simulink model "asbCubeSat"  (R2021a)
settings: Solver=FixedStepAuto  StartTime=0.0  StopTime=43200  FixedStep=CubeSatTimeStep  RelTol=1e-3  EnableMultiTasking=on
PreLoadFcn:
  | if ~builtin('license','test','Virtual_Reality_Toolbox')
  |     assignin('base','variantVisualization',0)
  | end
InitFcn:
  | if evalin('base', 'exist(''variantVisualization'',''var'')') && ...
  |         evalin('base', 'variantVisualization == 1')
  |     if ~builtin('license','checkout','Virtual_Reality_Toolbox')
  |         error(message('aeroblks_cubesat:cubesat:licenseFailAnim'));
  |     end
  | end
  | 
  | if ~evalin('base','exist(''CubeSatTimeStep'')')
  |     assignin('base','CubeSatTimeStep',5);
  | end
undefined symbols (not defined in the file): asbCubeSatEnvironmentLib, CubeSatTimeStep, Enviroment, IAU, initCond, km, s, vehicle
libraries: aerolibutil x17, sharedutil x6, aerolibconvert2 x4, aerolibtransform2 x1, aerolibcelestial x1, SignalEditorBlockLib x1, asbCubeSatSensorsLib x1, asbCubeSatDynamicsLib x1, aerolibobsolete x1, aerolibattitudesys x1, simulink x1, vrlib x1
settings Model: RequirementInfo={} %GIDa_aedc6be2_fb6a_446c_8c25_10b8bc9db182  SnapshotInterval=1  ExtModeAutoUpdateStatusClock=off  OrderedModelArguments=off  Creator=The MathWorks, Inc.  LastModifiedBy=noraw
settings SolverCC: AlgebraicLoopSolver=TrustRegion
settings DataIOCC: LimitDataPoints=on  SaveFormat=Array  SaveOutput=off  DSMLogging=off  SaveTime=off  ReturnWorkspaceOutputs=off
settings OptimizationCC: DefaultParameterBehavior=Inlined  OptimizeBlockIOStorage=off  BufferReuse=off  GlobalBufferReuse=off  ExpressionFolding=off  ExpressionDepthLimit=2147483647  LocalBlockOutputs=off  InitFltsAndDblsToZero=on  LifeSpan=inf  OptimizeDataStoreBuffers=off  BusAssignmentInplaceUpdate=off
settings DebuggingCC: SignalResolutionControl=TryResolveAllWithWarning  MultiTaskDSMMsg=warning  MultiTaskCondExecSysMsg=none  AssertControl=DisableAll  StateNameClashWarn=warning  PregeneratedLibrarySubsystemCodeDiagnostic=none  SFUnexpectedBacktrackingDiag=warning  SFNoUnconditionalDefaultTransitionDiag=warning  SFExecutionAtInitializationDiag=none  SFMachineParentedDataDiag=warning  ArithmeticOperatorsInVariantConditions=warning
settings HardwareCC: ProdBitPerPointer=32  ProdBitPerSizeT=32  ProdBitPerPtrDiffT=32  ProdLargestAtomicFloat=None  ProdIntDivRoundTo=Undefined  ProdEndianess=Unspecified  ProdWordSize=32  ProdHWDeviceType=32-bit Generic
settings ModelReferenceCC: UpdateModelReferenceTargets=IfOutOfDate  ModelReferenceMinAlgLoopOccurrences=on  PropagateSignalLabelsOutOfModel=off
settings SFSimCC: SimUseLocalCustomCode=off
settings RTWCC: RTWUseLocalCustomCode=off
settings CodeAppCC: StateflowObjectComments=on
settings GRTTargetCC: TargetFcnLib=ansi_tfl_tmw.mat  TargetLangStandard=C89/C90 (ANSI)  CombineOutputUpdateFcns=off  GRTInterface=on
settings ConfigComp: CovMetricSettings=dw  CovSaveCumulativeToWorkspaceVar=on  CovSaveSingleToWorkspaceVar=on  CovExternalEMLEnable=off

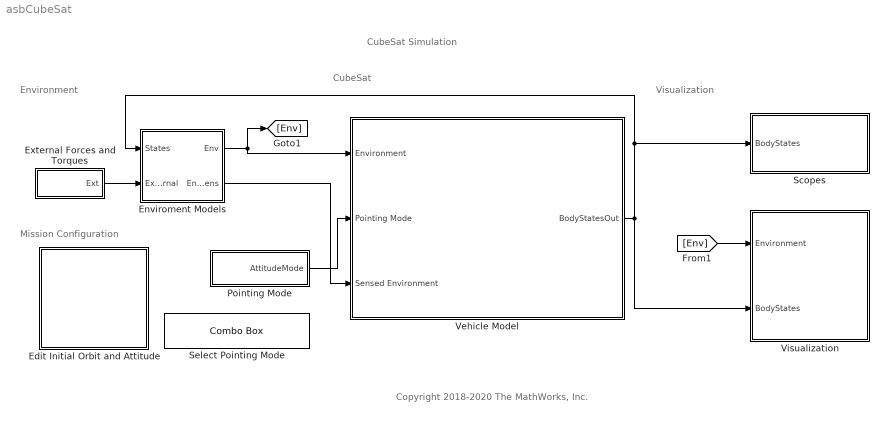
== system asbCubeSat ==
  note: Visualization
  note: CubeSat
  note: Environment
  note: Copyright 2018-2020 The MathWorks, Inc.
  note: CubeSat Simulation
  note: Mission Configuration
  Edit Initial Orbit and Attitude : Subsystem  mask(CubeSat Initial Conditions){sim_t0=2458488, epoch=2451545, method=Keplerian Orbital Elements, a=6786233.13, ecc=0.0010537, incl=51.7519, omega=95.2562, argp=93.4872, nu=302.9234, truelon=0, arglat=0, lonper=0, r_eci=[-2981784.257 5207055.9381 3161595.3068], v_eci=[-3384.4834 -4887.7595 4843.4609], r_ecef=[-5762650.9114 -1682704.282 3156028.2879], v_ecef=[3832.57 -4024.9014 4837.4311], lla=[27.88080034 -163.722102 408851.6223], v_ned=[5468.7396 4937.8129 -7.4627367], euler=[0 0 0], pqr=[0 0 -0.05168]}
      mask prompts: sim_t0 "spacecraft:cubesat:StartDate"; epoch "spacecraft:cubesat:ECIEpoch"; method "spacecraft:cubesat:InputMethod"; a "spacecraft:cubesat:SemiMajorAxis"; ecc "spacecraft:cubesat:Eccentricity"; incl "spacecraft:cubesat:Inclination"; omega "spacecraft:cubesat:RAAN"; argp "spacecraft:cubesat:ArgP"; nu "spacecraft:cubesat:TrueAnomaly"; truelon "spacecraft:cubesat:TrueLon"; arglat "spacecraft:cubesat:ArgLat"; lonper "spacecraft:cubesat:LonPer"; r_eci "spacecraft:cubesat:ECIPos"; v_eci "spacecraft:cubesat:ECIVel"; r_ecef "spacecraft:cubesat:ECEFPos"; v_ecef "spacecraft:cubesat:ECEFVel"; lla "spacecraft:cubesat:LLA"; v_ned "spacecraft:cubesat:NEDVel"; euler "spacecraft:cubesat:Euler"; pqr "spacecraft:cubesat:BodyAngRates"
      mask help: spacecraft:cubesat:InitCondBlockDesc
      mask init:
      | initCond = cubeSatCallback(gcb, 'computeIC', method, sim_t0, epoch, a, ecc, incl,...
      |     omega, argp, nu, truelon, arglat, lonper, r_eci, v_eci, r_ecef, v_ecef, lla,...
      |     v_ned, euler, pqr);
      mask TypeOptions method: spacecraft:cubesat:InputKeplerian | spacecraft:cubesat:InputECI | spacecraft:cubesat:InputECEF | spacecraft:cubesat:InputLLANED
      mask Callback method: cubeSatCallback(gcb, 'handleMethod');
      mask Callback ecc: cubeSatCallback(gcb, 'handleCircularOrbit');
      mask Callback incl: cubeSatCallback(gcb, 'handleCircularOrbit');
      mask DialogControl sim_t0 Prompt: Start date [Julian date]:
      mask DialogControl sim_t0 Tooltip: spacecraft:spacecraft:StartDateTT
      mask DialogControl icTab Prompt: spacecraft:cubesat:InitCond
      mask DialogControl epoch Prompt: Epoch of ECI frame [Julian date]:
      mask DialogControl epoch Tooltip: spacecraft:cubesat:ECIEpochTT
      mask DialogControl Container9 Prompt: spacecraft:cubesat:InitCondOrbit
      mask DialogControl method Prompt: Input method:
      mask DialogControl method Tooltip: spacecraft:cubesat:InputMethodTT
      mask DialogControl a Prompt: Semi-major axis [m]:
      mask DialogControl a Tooltip: spacecraft:cubesat:SemiMajorAxisTT
      mask DialogControl ecc Prompt: Eccentricity:
      mask DialogControl ecc Tooltip: spacecraft:cubesat:EccentricityTT
      mask DialogControl incl Prompt: Inclination [deg]:
      mask DialogControl incl Tooltip: spacecraft:cubesat:InclinationTT
      mask DialogControl omega Prompt: Right ascension of the ascending node [deg]:
      mask DialogControl omega Tooltip: spacecraft:cubesat:RAANTT
      mask DialogControl argp Prompt: Argument of periapsis [deg]:
      mask DialogControl argp Tooltip: spacecraft:cubesat:ArgPTT
      mask DialogControl nu Prompt: True anomaly [deg]:
      mask DialogControl nu Tooltip: spacecraft:cubesat:TrueAnomalyTT
      mask DialogControl truelon Prompt: True longitude [deg] (circular equatorial):
      mask DialogControl truelon Tooltip: spacecraft:cubesat:TrueLonTT
      mask DialogControl arglat Prompt: Argument of latitude [deg] (circular inclined):
      mask DialogControl arglat Tooltip: spacecraft:cubesat:ArgLatTT
      mask DialogControl lonper Prompt: Longitude of periapsis [deg] (elliptical equatorial):
      mask DialogControl lonper Tooltip: spacecraft:cubesat:LonPerTT
      mask DialogControl r_eci Prompt: ECI position vector [m]:
      mask DialogControl r_eci Tooltip: spacecraft:cubesat:ECIPosTT
      mask DialogControl v_eci Prompt: ECI velocity vector [m/s]:
      mask DialogControl v_eci Tooltip: spacecraft:cubesat:ECIVelTT
      mask DialogControl r_ecef Prompt: ECEF position vector [m]:
      mask DialogControl r_ecef Tooltip: spacecraft:cubesat:ECEFPosTT
      mask DialogControl v_ecef Prompt: ECEF velocity vector [m/s]:
      mask DialogControl v_ecef Tooltip: spacecraft:cubesat:ECEFVelTT
      mask DialogControl lla Prompt: Geodetic latitude, longitude, altitude [deg, deg, m]:
      mask DialogControl lla Tooltip: spacecraft:cubesat:LLATT
      mask DialogControl v_ned Prompt: NED velocity vector [m/s]:
      mask DialogControl v_ned Tooltip: spacecraft:cubesat:NEDVelTT
      mask DialogControl Container11 Prompt: spacecraft:cubesat:InitCondAttitude
      mask DialogControl euler Prompt: Initial Euler angles (roll, pitch, yaw) [deg]:
      mask DialogControl euler Tooltip: spacecraft:cubesat:EulerTT
      mask DialogControl pqr Prompt: Initial body angular rates [deg/s]:
      mask DialogControl pqr Tooltip: spacecraft:cubesat:BodyAngRatesTT
      mask Display:
      | text(.1, .9, [' a = ' sprintf('%.1f', str2double(get_param(gcb, 'a'))) ' m'],'horizontalAlignment','left','texmode','on');
      | text(.1, .75, [' e = ' get_param(gcb, 'ecc')],'horizontalAlignment','left','texmode', 'on')
      | text(.1, .6, ['  i = ' get_param(gcb, 'incl') '\circ'],'horizontalAlignment','left','texmode', 'on')
      | text(.1, .45, ['\Omega = ' get_param(gcb, 'omega') '\circ'],'horizontalAlignment','left','texmode', 'on')
      | text(.1, .3, ['\omega = ' get_param(gcb, 'argp') '\circ'],'horizontalAlignment','left','texmode', 'on')
      | text(.1, .15, [' \nu = ' get_param(gcb, 'nu') '\circ'],'horizontalAlignment','left','texmode', 'on')
  Enviroment Models : Subsystem  AncestorBlock=asbCubeSatEnvironmentLib/Enviroment
  "External Forces and Torques " : Subsystem
  Pointing Mode : Subsystem
  Scopes : Subsystem  VariantControl=visOff
  Select Pointing Mode : ComboBox  LabelPosition=Hide  SelectedLabel=Nadir Pointing (Earth)
      settings: Values={{'Standby', 'Nadir Pointing (Earth)', 'Sun Tracking', 'Custom Schedule'}, [0 1 2 3]}
  Vehicle Model : Subsystem
      mask Display: image('CubeSatVehicle.PNG');
  Visualization : Subsystem  Variant=on  mask(Set Animation Properties){visSampleTime=5, cubesatSize=2e5, showAntenna=on, antennaHeight=1e6, antennaHalfAngle=25}
      mask prompts: visSampleTime "spacecraft:cubesat:AnimSampleTime"; cubesatSize "spacecraft:cubesat:MdlSize"; showAntenna "spacecraft:cubesat:ShowCone"; antennaHeight "spacecraft:cubesat:ConeHeight"; antennaHalfAngle "spacecraft:cubesat:ConeAngle"
      mask help: spacecraft:cubesat:VisBlockDesc
      mask Callback showAntenna:
      | if evalin('base', 'exist(''variantVisualization'',''var'')') ...
      |     && evalin('base', 'variantVisualization == 1') ...
      |     && builtin('license','test','Virtual_Reality_Toolbox')
      | 
      |     enable = get_param(gcb,'MaskEnables');
      |     if strcmp(get_param(gcb, 'showAntenna'), 'off')
      |         enable(4:5) = {'off'};
      |     else
      |         enable(4:5) = {'on'};
      |     end
      |     set_param(gcb,'MaskEnables', enable);
      |     clear enable
      | end
      mask DialogControl vrOpenBtn Prompt: spacecraft:cubesat:AnimOpenBtn
      mask DialogControl vrOpenBtn Callback:
      | if builtin('license','checkout','Virtual_Reality_Toolbox')
      |     vrmfunc('FnOpen',getSimulinkBlockHandle([gcb '/Virtual Reality World/VR Sink']));
      | end
      mask DialogControl visSampleTime Prompt: Animation refresh rate:
      mask DialogControl visSampleTime Tooltip: spacecraft:cubesat:AnimSampleTimeTT
      mask DialogControl cubesatSize Prompt: CubeSat display size [m]:
      mask DialogControl cubesatSize Tooltip: spacecraft:cubesat:MdlSizeTT
      mask DialogControl Container3 Prompt: spacecraft:cubesat:AntennaPropArea
      mask DialogControl showAntenna Prompt: Show antenna cone in animation
      mask DialogControl showAntenna Tooltip: spacecraft:cubesat:ShowConeTT
      mask DialogControl antennaHeight Prompt: Antenna cone height [m]:
      mask DialogControl antennaHeight Tooltip: spacecraft:cubesat:ConeHeightTT
      mask DialogControl antennaHalfAngle Prompt: Antenna cone half angle [deg]:
      mask DialogControl antennaHalfAngle Tooltip: spacecraft:cubesat:ConeAngleTT
  wires:
  Enviroment Models/1(Env) -> Vehicle Model/1(Environment), [Env]
  "External Forces and Torques "/1(Ext) -> Enviroment Models/2(External)
  Vehicle Model/1(BodyStatesOut) -> Visualization/2(BodyStates), Scopes/1(BodyStates), Enviroment Models/1(States)
  Pointing Mode/1(AttitudeMode) -> Vehicle Model/2(Pointing Mode)
  [Env] -> Visualization/1(Environment)
  Enviroment Models/2(EnvSens) -> Vehicle Model/3(Sensed Environment)

== system asbCubeSat/Edit Initial Orbit and Attitude ==

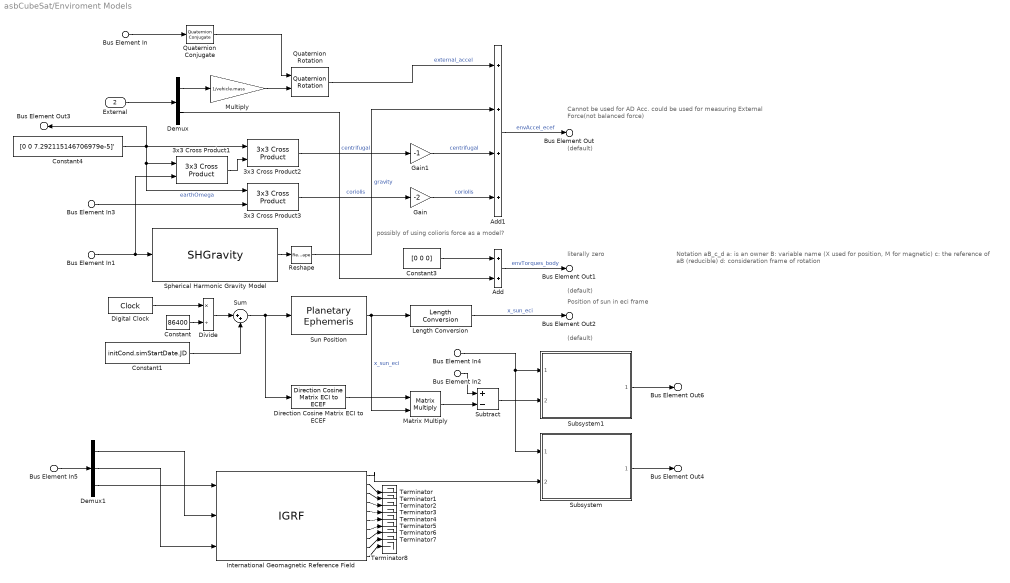
== system asbCubeSat/Enviroment Models ==
  note: (default)
  note: Notation
      | aB_c_d
      | a: is an owner
      | B: variable name (X used for position, M for magnetic)
      | c: the reference of aB (reducible)
      | d: consideration frame of rotation
  note: Cannot be used for AD
      | Acc. could be used for measuring External Force(not balanced force)
  note: literally zero
  note: Position of sun in eci frame
  note: (default)
  note: (default)
  note: possibly of using colioris force as a model?
  Bus Element In : Inport  PortName=States  Element=q_ecef2b
  Bus Element In4 : Inport  PortName=States  Element=q_ecef2b
  Bus Element In1 : Inport  PortName=States  Element=X_ecef
  Bus Element In2 : Inport  PortName=States  Element=X_ecef
  Bus Element In3 : Inport  PortName=States  Element=V_ecef
  Bus Element In5 : Inport  PortName=States  Element=LatLonAlt
  External : Inport  RequirementInfo={} %GIDa_966e36cb_16b5_4872_900e_7ca1bd630c23  Port=2
  3x3 Cross Product1 : sharedutil/3x3 Cross Product  aMode=aMode
      settings: SourceProductBaseCode=AE,PW,DR,MT,UV,VE
  3x3 Cross Product2 : sharedutil/3x3 Cross Product  aMode=aMode
      settings: SourceProductBaseCode=AE,PW,DR,MT,UV,VE
  3x3 Cross Product3 : sharedutil/3x3 Cross Product  aMode=aMode
      settings: SourceProductBaseCode=AE,PW,DR,MT,UV,VE
  Add : Sum  RequirementInfo={} %GIDa_1e3b988f_8e92_4de4_9735_9df8703148df
  Add1 : Sum  RequirementInfo={} %GIDa_b8d2c483_28a5_4509_a823_93e900185cc4  Inputs=++++
  Constant : Constant  Value=86400
  Constant1 : Constant  RequirementInfo={} %GIDa_d3dce1ea_7a4c_4489_9b49_860fce94c68a  Value=initCond.simStartDate.JD
  Constant3 : Constant  RequirementInfo={} %GIDa_08481c77_462d_49c1_8b19_5d7cc7c94401  Value=[0 0 0]
  Constant4 : Constant  Value=[0 0 7.292115146706979e-5]'
  Demux : Demux  RequirementInfo={} %GIDa_25e02362_af2f_4200_81e6_6d7271b48bfe  Outputs=2
  Demux1 : Demux  Outputs=3
  Digital Clock : DigitalClock  SampleTime=CubeSatTimeStep
  Direction Cosine Matrix ECI to ECEF : aerolibtransform2/Direction Cosine Matrix ECI to ECEF  red=IAU-2000/2006  year=2019  month=January  day=4  hour=0  min=0  sec=0  deltaT=Day  errorflag=Error  extraparamflag=off
      settings: AttributesFormatString=%<red>  SourceProductBaseCode=AE
  Divide : Product  Inputs=*/
  Gain : Gain  Gain=-2
  Gain1 : Gain  Gain=-1
  International Geomagnetic Reference Field : IGRF  time_in=off  month=January  day=4  year=2019
      settings: AttributesFormatString=%<generation>
  Length Conversion : aerolibconvert2/Length Conversion  IU=km  OU=m
  Matrix Multiply : Product  Multiplication=Matrix(*)
  Multiply : Gain  Gain=1/vehicle.mass
  Quaternion Conjugate : aerolibutil/Quaternion Conjugate
      settings: SourceProductBaseCode=AE
  Quaternion Rotation : aerolibutil/Quaternion Rotation
  Reshape : Reshape
  Spherical Harmonic Gravity Model : SHGravity  RequirementInfo={} %GIDa_e6b23945_77d7_4eed_b23b_331bed44acc0  degree=20  datafile='aerogmm2b.mat'
  Subsystem : Subsystem  ReferencedSubsystem=startNormEcef2Body
  Subsystem1 : Subsystem  ReferencedSubsystem=startNormEcef2Body
  Subtract : Sum  Inputs=+-
  Sum : Sum  Inputs=|++
  Sun Position : aerolibcelestial/Planetary Ephemeris  kmflag=km,km/s  epochflag=Julian date  de=DE421  nCenter=Earth  nTarget=Sun  errorflag=Error  velflag=off
      settings: SourceProductBaseCode=AE
  Terminator{,1..8} (9 alike) : Terminator
  Bus Element Out : Outport  VectorParamsAs1DForOutWhenUnconnected=off  PortName=Env  Element=envAccel_ecef
  Bus Element Out1 : Outport  VectorParamsAs1DForOutWhenUnconnected=off  PortName=Env  Element=envTorques_body
  Bus Element Out2 : Outport  VectorParamsAs1DForOutWhenUnconnected=off  PortName=Env  Element=x_sun_eci
  Bus Element Out3 : Outport  VectorParamsAs1DForOutWhenUnconnected=off  PortName=Env  Element=earthAngRate
  Bus Element Out6 : Outport  Port=2  PortName=EnvSens  Element=satS_body
  Bus Element Out4 : Outport  Port=2  PortName=EnvSens  Element=satM_body
  wires:
  Gain/1 -> Add1/4  "coriolis"
  Gain1/1 -> Add1/3  "centrifugal"
  3x3 Cross Product2/1 -> Gain1/1  "centrifugal"
  3x3 Cross Product3/1 -> Gain/1  "coriolis"
  Bus Element In3/1 -> 3x3 Cross Product3/2
  3x3 Cross Product1/1 -> 3x3 Cross Product2/2
  Reshape/1 -> Add1/2  "gravity"
  Quaternion Rotation/1 -> Add1/1  "external_accel"
  Quaternion Conjugate/1 -> Quaternion Rotation/1
  Multiply/1 -> Quaternion Rotation/2
  Constant1/1 -> Sum/2
  Divide/1 -> Sum/1
  Constant/1 -> Divide/2
  Length Conversion/1 -> Bus Element Out2/1  "x_sun_eci"
  Constant4/1 -> 3x3 Cross Product1/1, 3x3 Cross Product3/1, 3x3 Cross Product2/1, Bus Element Out3/1  "earthOmega"
  Sun Position/1 -> Matrix Multiply/2, Length Conversion/1  "x_sun_eci"
  Digital Clock/1 -> Divide/1
  Sum/1 -> Direction Cosine Matrix ECI to ECEF/1, Sun Position/1
  Spherical Harmonic Gravity Model/1 -> Reshape/1
  External/1 -> Demux/1
  Demux/2 -> Add/2
  Add/1 -> Bus Element Out1/1  "envTorques_body"
  Add1/1 -> Bus Element Out/1  "envAccel_ecef"
  Demux/1 -> Multiply/1
  Constant3/1 -> Add/1
  Bus Element In/1 -> Quaternion Conjugate/1
  Bus Element In1/1 -> Spherical Harmonic Gravity Model/1, 3x3 Cross Product1/2
  Direction Cosine Matrix ECI to ECEF/1 -> Matrix Multiply/1
  Matrix Multiply/1 -> Subtract/2
  Bus Element In2/1 -> Subtract/1
  Bus Element In5/1 -> Demux1/1
  Demux1/1 -> International Geomagnetic Reference Field/2
  Demux1/2 -> International Geomagnetic Reference Field/3
  Demux1/3 -> International Geomagnetic Reference Field/1
  Bus Element In4/1 -> Subsystem1/1, Subsystem/1
  International Geomagnetic Reference Field/1 -> Subsystem/2
  Subsystem/1 -> Bus Element Out4/1
  International Geomagnetic Reference Field/2 -> Terminator/1
  International Geomagnetic Reference Field/3 -> Terminator1/1
  International Geomagnetic Reference Field/4 -> Terminator2/1
  International Geomagnetic Reference Field/5 -> Terminator3/1
  International Geomagnetic Reference Field/6 -> Terminator4/1
  International Geomagnetic Reference Field/7 -> Terminator5/1
  International Geomagnetic Reference Field/8 -> Terminator6/1
  International Geomagnetic Reference Field/9 -> Terminator7/1
  International Geomagnetic Reference Field/10 -> Terminator8/1
  Subtract/1 -> Subsystem1/2
  Subsystem1/1 -> Bus Element Out6/1

== system asbCubeSat/External Forces and Torques  ==
  Forces_Body : Constant  Value=[0 0 0]
  Mux : Mux  RequirementInfo={} %GIDa_ef4ca723_4eef_40f8_bb1e_99de60d2b248  Inputs=2
  Torques_Body : Constant  Value=[0 0 0]
  Ext : Outport  RequirementInfo={} %GIDa_0f078eca_6127_499d_b81c_658503a40261  VectorParamsAs1DForOutWhenUnconnected=off
  wires:
  Forces_Body/1 -> Mux/1
  Torques_Body/1 -> Mux/2
  Mux/1 -> Ext/1

== system asbCubeSat/Pointing Mode ==
  note: Modes:
      | 0 = Off
      | 1 = Earth (Nadir)
      | 2 = Sun
  Mode : Constant  SampleTime=-1
  Multiport Switch : MultiPortSwitch  DataPortOrder=Specify indices  DataPortIndices={3, [0,1,2]}  DiagnosticForDefault=None
  Signal Editor : SignalEditorBlockLib/Signal Editor  FileName=SignalEditorPointing.mat  ActiveScenario=PointingScenario  ActiveSignal=PointingMode  IsBus=off  OutputBusObjectStr=Bus: BusObject  SampleTime=0  Interpolate=off  ZeroCross=off  OutputAfterFinalValue=Setting to zero  Unit=inherit  PreserveSignalName=on
  AttitudeMode : Outport  VectorParamsAs1DForOutWhenUnconnected=off
  wires:
  Signal Editor/1 -> Multiport Switch/2
  Mode/1 -> Multiport Switch/1, Multiport Switch/3
  Multiport Switch/1 -> AttitudeMode/1

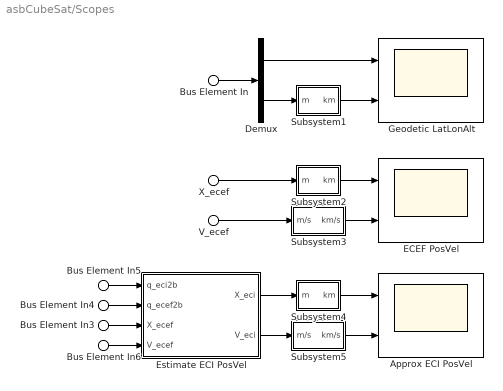
== system asbCubeSat/Scopes ==
  Bus Element In : Inport  PortName=BodyStates  Element=LatLonAlt
  X_ecef : Inport  PortName=BodyStates  Element=X_ecef
  Bus Element In3 : Inport  PortName=BodyStates  Element=X_ecef
  V_ecef : Inport  PortName=BodyStates  Element=V_ecef
  Bus Element In6 : Inport  PortName=BodyStates  Element=V_ecef
  Bus Element In4 : Inport  PortName=BodyStates  Element=q_ecef2b
  Bus Element In5 : Inport  PortName=BodyStates  Element=q_eci2b
  Approx ECI PosVel : Scope  NumInputPorts=2
  Demux : Demux  Outputs=[2 1]
  ECEF PosVel : Scope  NumInputPorts=2
  Estimate ECI PosVel : Subsystem
  Geodetic LatLonAlt : Scope  NumInputPorts=2
  Subsystem1 : Subsystem
  Subsystem2 : Subsystem
  Subsystem3 : Subsystem
  Subsystem4 : Subsystem
  Subsystem5 : Subsystem
  wires:
  Bus Element In/1 -> Demux/1
  Demux/1 -> Geodetic LatLonAlt/1
  Demux/2 -> Subsystem1/1(m)
  X_ecef/1 -> Subsystem2/1(m)
  V_ecef/1 -> Subsystem3/1(m/s)
  Estimate ECI PosVel/1(X_eci) -> Subsystem4/1(m)
  Estimate ECI PosVel/2(V_eci) -> Subsystem5/1(m/s)
  Bus Element In5/1 -> Estimate ECI PosVel/1(q_eci2b)
  Bus Element In4/1 -> Estimate ECI PosVel/2(q_ecef2b)
  Bus Element In3/1 -> Estimate ECI PosVel/3(X_ecef)
  Bus Element In6/1 -> Estimate ECI PosVel/4(V_ecef)
  Subsystem1/1(km) -> Geodetic LatLonAlt/2
  Subsystem2/1(km) -> ECEF PosVel/1
  Subsystem3/1(km/s) -> ECEF PosVel/2
  Subsystem4/1(km) -> Approx ECI PosVel/1
  Subsystem5/1(km/s) -> Approx ECI PosVel/2

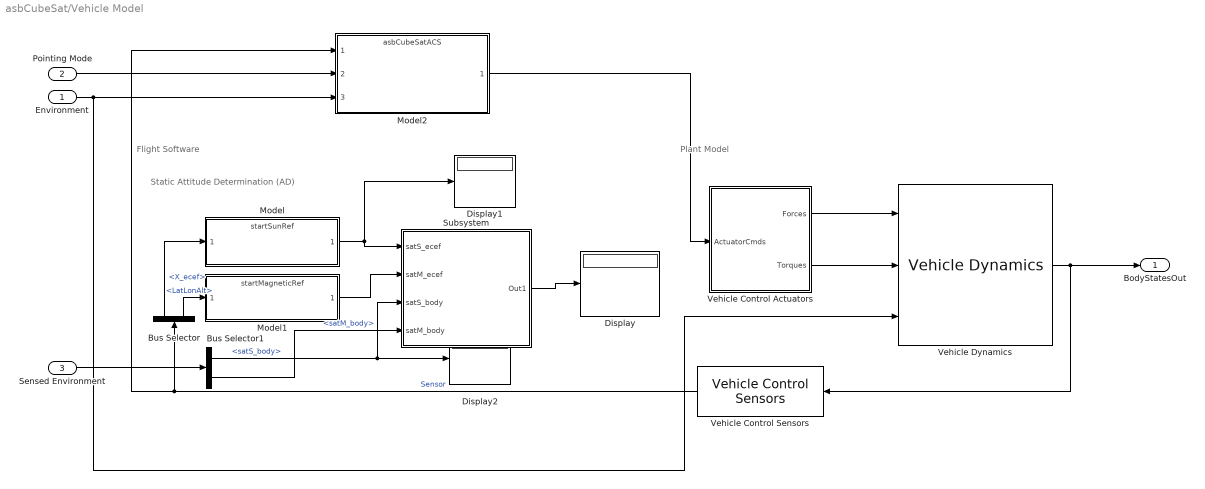
== system asbCubeSat/Vehicle Model ==
  note: Flight Software
  note: Plant Model
  note: Static Attitude Determination (AD)
  Environment : Inport
  Pointing Mode : Inport  Port=2
  Sensed Environment : Inport  Port=3
  Bus Selector : BusSelector  OutputSignals=X_ecef,LatLonAlt
  Bus Selector1 : BusSelector  OutputSignals=satS_body,satM_body
  Display : Display
  Display1 : Display
  Display2 : Display
  Model : ModelReference  ModelNameDialog=startSunRef.slx  SimulationMode=Normal  ModelReferenceVersion=1.6
  Model1 : ModelReference  ModelNameDialog=startMagneticRef.slx  SimulationMode=Normal  ModelReferenceVersion=1.5
  Model2 : ModelReference  ModelNameDialog=asbCubeSatACS.slx  SimulationMode=Normal  ModelReferenceVersion=4.0
  Subsystem : Subsystem
  Vehicle Control Actuators : Subsystem  AncestorBlock=asbCubeSatActuatorsLib/Vehicle Control Actuators
  Vehicle Control Sensors : asbCubeSatSensorsLib/Vehicle Control Sensors  SystemSampleTime=-1  VariantActivationTime=update diagram  Latency=0  AutoFrameSizeCalculation=off
  Vehicle Dynamics : asbCubeSatDynamicsLib/Vehicle Dynamics  SystemSampleTime=-1  VariantActivationTime=update diagram  Latency=0  AutoFrameSizeCalculation=off
  BodyStatesOut : Outport  OutDataTypeStr=Bus: StatesOutBus  VectorParamsAs1DForOutWhenUnconnected=off
  wires:
  Vehicle Dynamics/1 -> Vehicle Control Sensors/1, BodyStatesOut/1
  Pointing Mode/1 -> Model2/2
  Vehicle Control Actuators/1(" Forces") -> Vehicle Dynamics/1
  Vehicle Control Actuators/2(" Torques") -> Vehicle Dynamics/2
  Environment/1 -> Vehicle Dynamics/3, Model2/3
  Vehicle Control Sensors/1 -> Bus Selector/1, Model2/1  "Sensor"
  Bus Selector/2 -> Model1/1  "<LatLonAlt>"
  Bus Selector/1 -> Model/1  "<X_ecef>"
  Bus Selector1/1 -> Subsystem/3(satS_body), Display2/1  "<satS_body>"
  Bus Selector1/2 -> Subsystem/4(satM_body)  "<satM_body>"
  Model1/1 -> Subsystem/2(satM_ecef)
  Model/1 -> Subsystem/1(satS_ecef), Display1/1
  Subsystem/1(Out1) -> Display/1
  Model2/1 -> Vehicle Control Actuators/1(ActuatorCmds)
  Sensed Environment/1 -> Bus Selector1/1

== system asbCubeSat/Visualization ==
  Environment : Inport
  BodyStates : Inport  RequirementInfo={} %GIDa_d1e0371a_f352_4707_a071_6ff04189e700  Port=2
  No Visualization : Subsystem  VariantControl=visOff
  Virtual Reality World : Subsystem  VariantControl=visSL3D

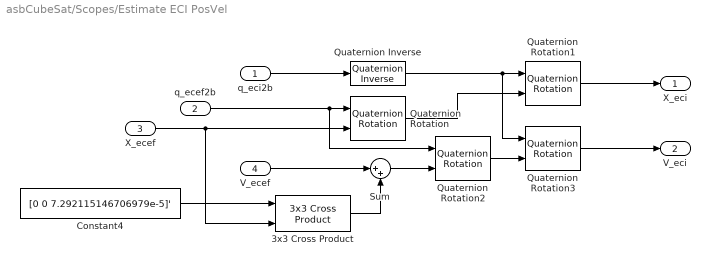
== system asbCubeSat/Scopes/Estimate ECI PosVel ==
  q_eci2b : Inport
  q_ecef2b : Inport  Port=2
  X_ecef : Inport  Port=3
  V_ecef : Inport  Port=4
  3x3 Cross Product : sharedutil/3x3 Cross Product  aMode=aMode
      settings: SourceProductBaseCode=AE,PW,DR,MT,UV,VE
  Constant4 : Constant  Value=[0 0 7.292115146706979e-5]'
  Quaternion Inverse : aerolibutil/Quaternion Inverse
  Quaternion Rotation{,1..3} (4 alike) : aerolibutil/Quaternion Rotation
  Sum : Sum  Inputs=|++
  X_eci : Outport  VectorParamsAs1DForOutWhenUnconnected=off
  V_eci : Outport  Port=2  VectorParamsAs1DForOutWhenUnconnected=off
  wires:
  Sum/1 -> Quaternion Rotation2/2
  3x3 Cross Product/1 -> Sum/2
  V_ecef/1 -> Sum/1
  Quaternion Rotation/1 -> Quaternion Rotation1/2
  q_ecef2b/1 -> Quaternion Rotation/1, Quaternion Rotation2/1
  Quaternion Inverse/1 -> Quaternion Rotation3/1, Quaternion Rotation1/1
  Constant4/1 -> 3x3 Cross Product/1
  Quaternion Rotation2/1 -> Quaternion Rotation3/2
  q_eci2b/1 -> Quaternion Inverse/1
  Quaternion Rotation1/1 -> X_eci/1
  X_ecef/1 -> 3x3 Cross Product/2, Quaternion Rotation/2
  Quaternion Rotation3/1 -> V_eci/1

== system asbCubeSat/Scopes/Subsystem1 ==
  m : Inport  Unit=m
  Unit Conversion : UnitConversion
  km : Outport  Unit=km  VectorParamsAs1DForOutWhenUnconnected=off
  wires:
  m/1 -> Unit Conversion/1
  Unit Conversion/1 -> km/1

== system asbCubeSat/Scopes/Subsystem2 ==
  m : Inport  Unit=m
  Unit Conversion : UnitConversion
  km : Outport  Unit=km  VectorParamsAs1DForOutWhenUnconnected=off
  wires:
  Unit Conversion/1 -> km/1
  m/1 -> Unit Conversion/1

== system asbCubeSat/Scopes/Subsystem3 ==
  m/s : Inport  Unit=m/s
  Unit Conversion : UnitConversion
  km/s : Outport  Unit=km/s  VectorParamsAs1DForOutWhenUnconnected=off
  wires:
  m/s/1 -> Unit Conversion/1
  Unit Conversion/1 -> km/s/1

== system asbCubeSat/Scopes/Subsystem4 ==
  m : Inport  Unit=m
  Unit Conversion : UnitConversion
  km : Outport  Unit=km  VectorParamsAs1DForOutWhenUnconnected=off
  wires:
  Unit Conversion/1 -> km/1
  m/1 -> Unit Conversion/1

== system asbCubeSat/Scopes/Subsystem5 ==
  m/s : Inport  Unit=m/s
  Unit Conversion : UnitConversion
  km/s : Outport  Unit=km/s  VectorParamsAs1DForOutWhenUnconnected=off
  wires:
  m/s/1 -> Unit Conversion/1
  Unit Conversion/1 -> km/s/1

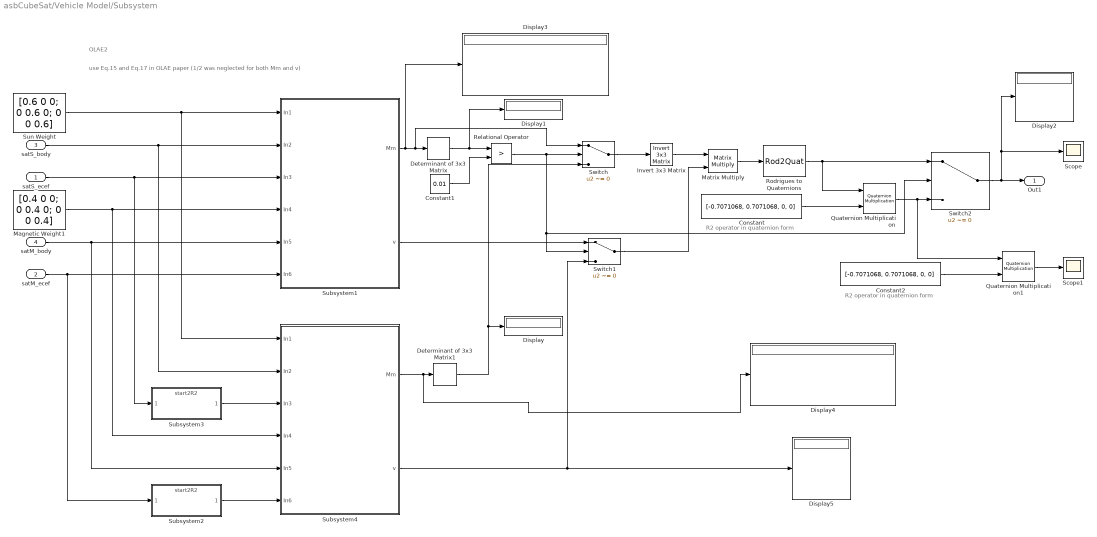
== system asbCubeSat/Vehicle Model/Subsystem ==
  note: R2 operator in quaternion form
  note: OLAE2
  note: use Eq.15 and Eq.17 in OLAE paper (1/2 was neglected for both Mm and v)
  note: R2 operator in quaternion form
  satS_ecef : Inport  PortDimensions=3
  satM_ecef : Inport  Port=2  PortDimensions=3
  satS_body : Inport  Port=3  PortDimensions=3
  satM_body : Inport  Port=4  PortDimensions=3
  Constant : Constant  Value=[-0.7071068, 0.7071068, 0, 0]
  Constant1 : Constant  Value=0.01
  Constant2 : Constant  Value=[-0.7071068, 0.7071068, 0, 0]
  Determinant of 3x3 Matrix : sharedutil/Determinant of 3x3 Matrix  aMode=aMode
      settings: SourceProductBaseCode=AE,PW,DR,MT,UV,VE
  Determinant of 3x3 Matrix1 : sharedutil/Determinant of 3x3 Matrix  aMode=aMode
      settings: SourceProductBaseCode=AE,PW,DR,MT,UV,VE
  Display{,1..5} (6 alike) : Display
  Invert 3x3 Matrix : aerolibutil/Invert  3x3 Matrix
  Magnetic Weight1 : Constant  Value=[0.4 0 0; 0 0.4 0; 0 0 0.4]
  Matrix Multiply : Product  Multiplication=Matrix(*)
  Quaternion Multiplication : aerolibutil/Quaternion Multiplication
  Quaternion Multiplication1 : aerolibutil/Quaternion Multiplication
  Relational Operator : RelationalOperator  Operator=>  OutDataTypeStr=boolean  RndMeth=Simplest
  Rodrigues to Quaternions : Rod2Quat
  Scope : Scope
  Scope1 : Scope
  Subsystem1 : Subsystem
  Subsystem2 : ModelReference  ModelNameDialog=start2R2  SimulationMode=Normal  ModelReferenceVersion=3.23
  Subsystem3 : ModelReference  ModelNameDialog=start2R2  SimulationMode=Normal  ModelReferenceVersion=3.23
  Subsystem4 : Subsystem
  Sun Weight : Constant  Value=[0.6 0 0; 0 0.6 0; 0 0 0.6]
  Switch : Switch  Criteria=u2 ~= 0  ZeroCross=off
  Switch1 : Switch  Criteria=u2 ~= 0  ZeroCross=off
  Switch2 : Switch  Criteria=u2 ~= 0
  Out1 : Outport
  wires:
  Subsystem3/1 -> Subsystem4/3(In3)
  Invert 3x3 Matrix/1 -> Matrix Multiply/1
  Switch2/1 -> Scope/1, Display2/1, Out1/1
  satM_ecef/1 -> Subsystem1/6(In6), Subsystem2/1
  satM_body/1 -> Subsystem4/5(In5), Subsystem1/5(In5)
  Relational Operator/1 -> Switch/2, Switch1/2, Switch2/2
  satS_ecef/1 -> Subsystem1/3(In3), Subsystem3/1
  Subsystem4/1(Mm) -> Display4/1, Determinant of 3x3 Matrix1/1
  Switch/1 -> Invert 3x3 Matrix/1
  Magnetic Weight1/1 -> Subsystem4/4(In4), Subsystem1/4(In4)
  satS_body/1 -> Subsystem4/2(In2), Subsystem1/2(In2)
  Subsystem1/1(Mm) -> Display3/1, Switch/1, Determinant of 3x3 Matrix/1
  Sun Weight/1 -> Subsystem4/1(In1), Subsystem1/1(In1)
  Determinant of 3x3 Matrix1/1 -> Display/1, Switch/3
  Determinant of 3x3 Matrix/1 -> Relational Operator/1, Display1/1
  Subsystem1/2(v) -> Switch1/1
  Constant1/1 -> Relational Operator/2
  Constant/1 -> Quaternion Multiplication/2
  Subsystem4/2(v) -> Display5/1, Switch1/3
  Subsystem2/1 -> Subsystem4/6(In6)
  Matrix Multiply/1 -> Rodrigues to Quaternions/1
  Switch1/1 -> Matrix Multiply/2
  Rodrigues to Quaternions/1 -> Switch2/1, Quaternion Multiplication/1
  Quaternion Multiplication/1 -> Quaternion Multiplication1/1, Switch2/3
  Constant2/1 -> Quaternion Multiplication1/2
  Quaternion Multiplication1/1 -> Scope1/1

== system asbCubeSat/Vehicle Model/Vehicle Control Actuators ==
  ActuatorCmds : Inport  RequirementInfo={} %GIDa_020f38c4_9e26_4002_9065_5d46819fcfcb
  CubeSat Perfect Actuators : Subsystem  AncestorBlock=asbCubeSatActuatorsLib/CubeSat Perfect Actuators
  " Forces" : Outport  RequirementInfo={} %GIDa_e46e2c30_d205_4036_910c_a099c6c54d17  VectorParamsAs1DForOutWhenUnconnected=off
  " Torques" : Outport  RequirementInfo={} %GIDa_67b5453a_f72e_4aa8_be3c_a57a924d68da  Port=2  VectorParamsAs1DForOutWhenUnconnected=off
  wires:
  CubeSat Perfect Actuators/1(ForcesActual) -> " Forces"/1
  CubeSat Perfect Actuators/2(TorquesActual) -> " Torques"/1
  ActuatorCmds/1 -> CubeSat Perfect Actuators/1(Input)

== system asbCubeSat/Visualization/No Visualization ==
  BodyStates : Inport
  Environment : Inport  Port=2
  Terminator2 : Terminator
      settings: RequirementInfo={} %GIDa_803f6fff_5423_4e6f_a9df_7d3b0fb0a1d4
  Terminator3 : Terminator
      settings: RequirementInfo={} %GIDa_5d360e88_5b3d_45e7_ae99_5d46a57676c9
  wires:
  Environment/1 -> Terminator2/1
  BodyStates/1 -> Terminator3/1

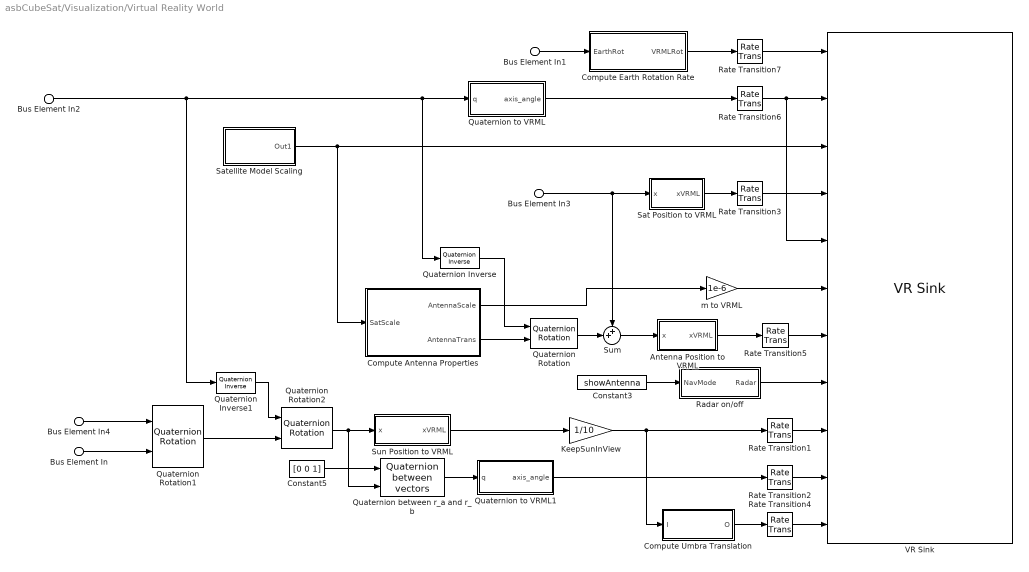
== system asbCubeSat/Visualization/Virtual Reality World ==
  Bus Element In3 : Inport  PortName=BodyStates  Element=X_ecef
  Bus Element In2 : Inport  PortName=BodyStates  Element=q_ecef2b
  Bus Element In4 : Inport  PortName=BodyStates  Element=q_eci2b
  Bus Element In : Inport  Port=2  PortName=Environment  Element=x_sun_eci
  Bus Element In1 : Inport  Port=2  PortName=Environment  Element=earthAngRate
  Antenna Position to VRML : Subsystem
  Compute Antenna Properties : Subsystem
  Compute Earth Rotation Rate : Subsystem
  Compute Umbra Translation : Subsystem
  Constant3 : Constant  Value=showAntenna
  Constant5 : Constant  Value=[0 0 1]
  KeepSunInView : Gain  Gain=1/10
  Quaternion Inverse : aerolibutil/Quaternion Inverse
  Quaternion Inverse1 : aerolibutil/Quaternion Inverse
  Quaternion Rotation : aerolibutil/Quaternion Rotation
  Quaternion Rotation1 : aerolibutil/Quaternion Rotation
  Quaternion Rotation2 : aerolibutil/Quaternion Rotation
  Quaternion between r_a and r_b : aerolibattitudesys/Quaternion between vectors
      settings: SourceProductBaseCode=AE
  Quaternion to VRML : Subsystem
  Quaternion to VRML1 : Subsystem
  Radar on/off : Subsystem
  Rate Transition{1..7} (7 alike) : RateTransition
  Sat Position to VRML : Subsystem
  Satellite Model Scaling : Subsystem
  Sum : Sum  Inputs=++|
  Sun Position to VRML : Subsystem
  VR Sink : vrlib/VR Sink  InstantiateOnLoad=on  SampleTime=visSampleTime  ViewEnable=on  RemoteChange=off  RemoteView=off  FieldsWritten=Earth.rotation.4.1.1.double#Satellite.rotation.4.1.1.double#Satellite.scale.3.1.1.double#Satellite.translation.3.1.1.double#AntennaCone.rotation.4.1.1.double#AntennaCone.scale.3.1.1.double#AntennaCone.translation.3.1.1.double#AntennaMaterial.transparency.1.1.1.double#Sun.translation.3.1.1.double#Umbra.rotation.4.1.1.double#Umbra.translation.3.1.1.double  WorldFileName=cubesatAnim.wrl  WorldDescription=CubeSat Orbit Animation  AutoView=on  VideoDimensions=[]  AllowVariableSize=off  FigureProperties="{'Position', 'Name', 'Viewpoint', 'CameraBound', 'CameraDirection', 'CameraPosition', 'CameraUpVector', 'ZoomFactor', 'Antialiasing', 'Headlight', 'Lighting', 'NavPanel', 'Sound', 'StatusBar', 'Stereo3D', 'Stereo3DCameraOffset', 'Stereo3DHIT', 'ToolBar', 'Textures', 'Transparency', 'Triad', 'Wireframe', 'NavZones', 'NavMode', 'NavSpeed', 'CaptureFileFormat', 'CaptureFileName', 'Record2DCompressMethod', 'Record2DCompressQuality', 'Record2D', 'Record2DFileName', 'Record2DFPS'; [5.9460000000000002e+02   1.9899999999999989e+02   7.9200000000000000e+02   5.2680000000000007e+02], 'CubeSat Orbit Animation', 'EarthSide', 'on', [-1.2074750837207472e-01   4.7652371552860603e-02  -9.9153884982249374e-01], [2.6564451841856895e+00  -1.0483521741629542e+00  -1.8614530390514616e-01], [-7.5307534652544389e-02   9.9552904182351576e-01   5.7014928838841489e-02], [1.0000000000000000e+00], 'on', 'on', 'on', 'halfbar', 'on', 'on', 'off', [1.0000000149011612e-01], [0.0000000000000000e+00], 'on', 'on', 'on', 'none', 'off', 'off', 'examine', 'normal', 'tif', '%f_anim_%n.tif', 'auto', [7.5000000000000000e+01], 'off', '%f_anim_%n.avi', 'auto'}"
  m to VRML : Gain  Gain=1e-6
  wires:
  Bus Element In2/1 -> Quaternion to VRML/1(q), Quaternion Inverse/1, Quaternion Inverse1/1
  Constant3/1 -> Radar on/off/1(NavMode)
  Bus Element In3/1 -> Sat Position to VRML/1(x), Sum/1
  Quaternion Inverse/1 -> Quaternion Rotation/1
  Sum/1 -> Antenna Position to VRML/1(x)
  Quaternion Rotation/1 -> Sum/2
  Quaternion Rotation2/1 -> Sun Position to VRML/1(x), Quaternion between r_a and r_b/2
  Quaternion Rotation1/1 -> Quaternion Rotation2/2
  Quaternion Inverse1/1 -> Quaternion Rotation2/1
  Sun Position to VRML/1(xVRML) -> KeepSunInView/1
  Quaternion between r_a and r_b/1 -> Quaternion to VRML1/1(q)
  Constant5/1 -> Quaternion between r_a and r_b/1
  m to VRML/1 -> VR Sink/6
  Antenna Position to VRML/1(xVRML) -> Rate Transition5/1
  Compute Earth Rotation Rate/1(VRMLRot) -> Rate Transition7/1
  Sat Position to VRML/1(xVRML) -> Rate Transition3/1
  Radar on/off/1(Radar) -> VR Sink/8
  Quaternion to VRML1/1(axis_angle) -> Rate Transition2/1
  KeepSunInView/1 -> Compute Umbra Translation/1(I), Rate Transition1/1
  Compute Umbra Translation/1(O) -> Rate Transition4/1
  Satellite Model Scaling/1(Out1) -> VR Sink/3, Compute Antenna Properties/1(SatScale)
  Compute Antenna Properties/1(AntennaScale) -> m to VRML/1
  Compute Antenna Properties/2(AntennaTrans) -> Quaternion Rotation/2
  Bus Element In4/1 -> Quaternion Rotation1/1
  Bus Element In/1 -> Quaternion Rotation1/2
  Rate Transition4/1 -> VR Sink/11
  Rate Transition1/1 -> VR Sink/9
  Rate Transition2/1 -> VR Sink/10
  Bus Element In1/1 -> Compute Earth Rotation Rate/1(EarthRot)
  Rate Transition7/1 -> VR Sink/1
  Rate Transition3/1 -> VR Sink/4
  Rate Transition5/1 -> VR Sink/7
  Quaternion to VRML/1(axis_angle) -> Rate Transition6/1
  Rate Transition6/1 -> VR Sink/5, VR Sink/2

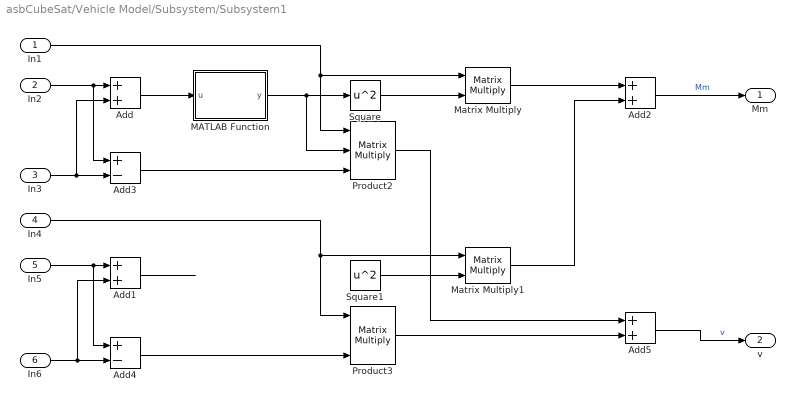
== system asbCubeSat/Vehicle Model/Subsystem/Subsystem1 ==
  In1 : Inport  PortDimensions=[3 3]
  In2 : Inport  Port=2  PortDimensions=3
  In3 : Inport  Port=3  PortDimensions=3
  In4 : Inport  Port=4  PortDimensions=[3 3]
  In5 : Inport  Port=5  PortDimensions=3
  In6 : Inport  Port=6  PortDimensions=3
  Add{,1..2,5} (4 alike) : Sum
  Add3 : Sum  Inputs=+-
  Add4 : Sum  Inputs=+-
  MATLAB Function : MATLAB Function  TreatAsAtomicUnit=on
  Matrix Multiply : Product  Multiplication=Matrix(*)
  Matrix Multiply1 : Product  Multiplication=Matrix(*)
  Product2 : Product  Inputs=3  Multiplication=Matrix(*)
  Product3 : Product  Inputs=3  Multiplication=Matrix(*)
  Square : Math  Operator=square  SaturateOnIntegerOverflow=on
  Square1 : Math  Operator=square  SaturateOnIntegerOverflow=on
  Mm : Outport
  v : Outport  Port=2
  wires:
  Add3/1 -> Product2/3
  In3/1 -> Add3/2, Add/2
  Add5/1 -> v/1  "v"
  Add2/1 -> Mm/1  "Mm"
  In1/1 -> Matrix Multiply/1, Product2/1
  Add4/1 -> Product3/3
  In2/1 -> Add3/1, Add/1
  Square1/1 -> Matrix Multiply1/2
  In5/1 -> Add4/1, Add1/1
  Matrix Multiply/1 -> Add2/1
  MATLAB Function/1(y) -> Product2/2, Square/1
  Matrix Multiply1/1 -> Add2/2
  Add1/1 -> ?
  Product2/1 -> Add5/1
  In6/1 -> Add1/2, Add4/2
  Product3/1 -> Add5/2
  ? -> Product3/2, Square1/1
  Square/1 -> Matrix Multiply/2
  In4/1 -> Matrix Multiply1/1, Product3/1
  Add/1 -> MATLAB Function/1(u)

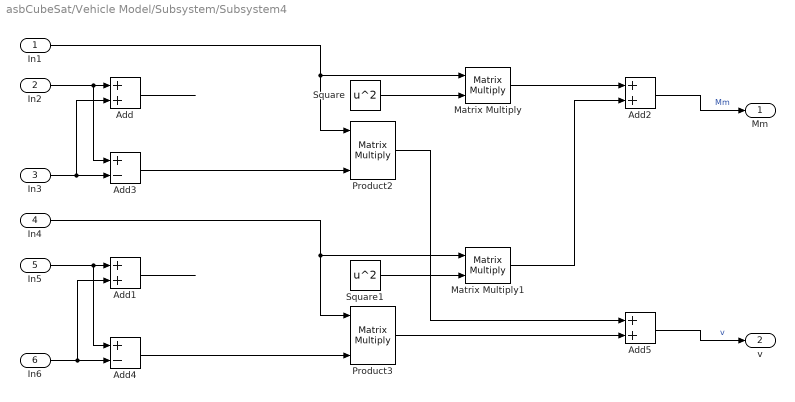
== system asbCubeSat/Vehicle Model/Subsystem/Subsystem4 ==
  In1 : Inport  PortDimensions=[3 3]
  In2 : Inport  Port=2  PortDimensions=3
  In3 : Inport  Port=3  PortDimensions=3
  In4 : Inport  Port=4  PortDimensions=[3 3]
  In5 : Inport  Port=5  PortDimensions=3
  In6 : Inport  Port=6  PortDimensions=3
  Add{,1..2,5} (4 alike) : Sum
  Add3 : Sum  Inputs=+-
  Add4 : Sum  Inputs=+-
  Matrix Multiply : Product  Multiplication=Matrix(*)
  Matrix Multiply1 : Product  Multiplication=Matrix(*)
  Product2 : Product  Inputs=3  Multiplication=Matrix(*)
  Product3 : Product  Inputs=3  Multiplication=Matrix(*)
  Square : Math  Operator=square  SaturateOnIntegerOverflow=on
  Square1 : Math  Operator=square  SaturateOnIntegerOverflow=on
  Mm : Outport
  v : Outport  Port=2
  wires:
  Add3/1 -> Product2/3
  In3/1 -> Add3/2, Add/2
  Add5/1 -> v/1  "v"
  Add2/1 -> Mm/1  "Mm"
  In1/1 -> Matrix Multiply/1, Product2/1
  Add4/1 -> Product3/3
  In2/1 -> Add3/1, Add/1
  Square1/1 -> Matrix Multiply1/2
  In5/1 -> Add4/1, Add1/1
  Matrix Multiply/1 -> Add2/1
  ? -> Product2/2, Square/1
  Matrix Multiply1/1 -> Add2/2
  Add1/1 -> ?
  Product2/1 -> Add5/1
  In6/1 -> Add1/2, Add4/2
  Product3/1 -> Add5/2
  ? -> Product3/2, Square1/1
  Square/1 -> Matrix Multiply/2
  In4/1 -> Matrix Multiply1/1, Product3/1
  Add/1 -> ?

== system asbCubeSat/Vehicle Model/Vehicle Control Actuators/CubeSat Perfect Actuators ==
  Input : Inport
  Bus Selector : BusSelector  OutputSignals=TorqueCmds
  Constant : Constant  Value=[0 0 0]
  Gain : Gain
  ForcesActual : Outport  VectorParamsAs1DForOutWhenUnconnected=off
  TorquesActual : Outport  Port=2  VectorParamsAs1DForOutWhenUnconnected=off
  wires:
  Constant/1 -> ForcesActual/1  "forcesAct"
  Gain/1 -> TorquesActual/1  "torquesAct"
  Bus Selector/1 -> Gain/1  "<TorqueCmds>"
  Input/1 -> Bus Selector/1  "ActuatorCmds"

== system asbCubeSat/Visualization/Virtual Reality World/Antenna Position to VRML ==
  x : Inport
  ECEF to VRML : Subsystem
  Length Conversion : aerolibconvert2/Length Conversion  IU=m  OU=km
  km to VRML units : Gain  Gain=1/1000
  xVRML : Outport  VectorParamsAs1DForOutWhenUnconnected=off
  wires:
  Length Conversion/1 -> km to VRML units/1
  km to VRML units/1 -> ECEF to VRML/1(M)
  x/1 -> Length Conversion/1
  ECEF to VRML/1(VR) -> xVRML/1

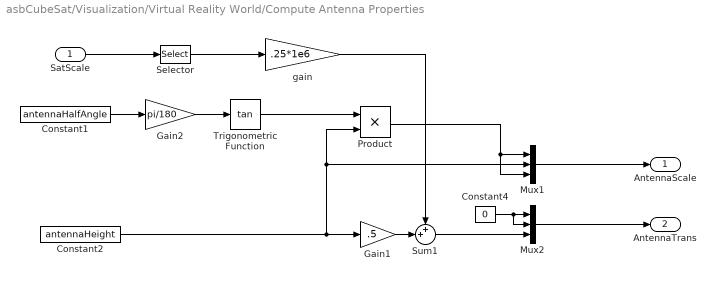
== system asbCubeSat/Visualization/Virtual Reality World/Compute Antenna Properties ==
  SatScale : Inport
  Constant1 : Constant  Value=antennaHalfAngle
  Constant2 : Constant  Value=antennaHeight
  Constant4 : Constant  Value=0
  Gain1 : Gain  Gain=.5
  Gain2 : Gain  Gain=pi/180
  Mux1 : Mux  Inputs=3
  Mux2 : Mux  Inputs=3
  Product : Product
  Selector : Selector  InputPortWidth=3  IndexOptions=Index vector (dialog)  Indices=1  OutputSizes=1
  Sum1 : Sum  Inputs=++|
  Trigonometric Function : Trigonometry  Operator=tan
  gain : Gain  Gain=.25*1e6
  AntennaScale : Outport  VectorParamsAs1DForOutWhenUnconnected=off
  AntennaTrans : Outport  Port=2  VectorParamsAs1DForOutWhenUnconnected=off
  wires:
  Gain2/1 -> Trigonometric Function/1
  Constant4/1 -> Mux2/1, Mux2/2
  Sum1/1 -> Mux2/3
  Constant2/1 -> Gain1/1, Mux1/2, Product/2
  gain/1 -> Sum1/1
  Constant1/1 -> Gain2/1
  Product/1 -> Mux1/3, Mux1/1
  Gain1/1 -> Sum1/2
  Trigonometric Function/1 -> Product/1
  Mux2/1 -> AntennaTrans/1
  Mux1/1 -> AntennaScale/1
  SatScale/1 -> Selector/1
  Selector/1 -> gain/1

== system asbCubeSat/Visualization/Virtual Reality World/Compute Earth Rotation Rate ==
  EarthRot : Inport
  Euler Angles to Quaternions : aerolibobsolete/Euler Angles to Quaternions
      settings: SourceProductBaseCode=AE
  Quaternion to VRML : Subsystem
  Sum : Sum  Inputs=|++
  Unit Delay : UnitDelay  SampleTime=-1  HasFrameUpgradeWarning=on
  VRMLRot : Outport  VectorParamsAs1DForOutWhenUnconnected=off
  wires:
  EarthRot/1 -> Sum/1
  Unit Delay/1 -> Sum/2
  Sum/1 -> Unit Delay/1, Euler Angles to Quaternions/1
  Euler Angles to Quaternions/1 -> Quaternion to VRML/1(q)
  Quaternion to VRML/1(AxisAngle) -> VRMLRot/1

== system asbCubeSat/Visualization/Virtual Reality World/Compute Umbra Translation ==
  I : Inport
  Add : Sum
  ConeHalfLength : Gain  Gain=692
  InvertSunPosECEF : Gain  Gain=-1
  unitVec : Subsystem
  O : Outport  VectorParamsAs1DForOutWhenUnconnected=off
  wires:
  ConeHalfLength/1 -> Add/2
  I/1 -> InvertSunPosECEF/1
  Add/1 -> O/1
  InvertSunPosECEF/1 -> unitVec/1(I), Add/1
  unitVec/1(O) -> ConeHalfLength/1

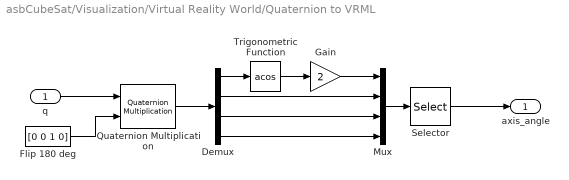
== system asbCubeSat/Visualization/Virtual Reality World/Quaternion to VRML ==
  q : Inport
  Demux : Demux
  Flip 180 deg : Constant  Value=[0 0 1 0]
  Gain : Gain  Gain=2
  Mux : Mux
  Quaternion Multiplication : aerolibutil/Quaternion Multiplication
  Selector : Selector  InputPortWidth=4  IndexOptions=Index vector (dialog)  Indices=[3 4 2 1]  OutputSizes=1
  Trigonometric Function : Trigonometry  Operator=acos
  axis_angle : Outport  VectorParamsAs1DForOutWhenUnconnected=off
  wires:
  Demux/4 -> Mux/4
  Demux/3 -> Mux/3
  Demux/2 -> Mux/2
  Gain/1 -> Mux/1
  Selector/1 -> axis_angle/1
  q/1 -> Quaternion Multiplication/1
  Mux/1 -> Selector/1
  Trigonometric Function/1 -> Gain/1
  Demux/1 -> Trigonometric Function/1
  Flip 180 deg/1 -> Quaternion Multiplication/2
  Quaternion Multiplication/1 -> Demux/1

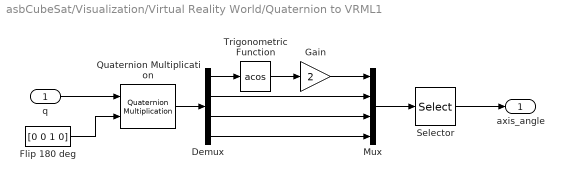
== system asbCubeSat/Visualization/Virtual Reality World/Quaternion to VRML1 ==
  q : Inport
  Demux : Demux
  Flip 180 deg : Constant  Value=[0 0 1 0]
  Gain : Gain  Gain=2
  Mux : Mux
  Quaternion Multiplication : aerolibutil/Quaternion Multiplication
  Selector : Selector  InputPortWidth=4  IndexOptions=Index vector (dialog)  Indices=[3 4 2 1]  OutputSizes=1
  Trigonometric Function : Trigonometry  Operator=acos
  axis_angle : Outport  VectorParamsAs1DForOutWhenUnconnected=off
  wires:
  Demux/4 -> Mux/4
  Demux/3 -> Mux/3
  Demux/2 -> Mux/2
  Gain/1 -> Mux/1
  Selector/1 -> axis_angle/1
  Mux/1 -> Selector/1
  Trigonometric Function/1 -> Gain/1
  Demux/1 -> Trigonometric Function/1
  Flip 180 deg/1 -> Quaternion Multiplication/2
  q/1 -> Quaternion Multiplication/1
  Quaternion Multiplication/1 -> Demux/1

== system asbCubeSat/Visualization/Virtual Reality World/Radar on//off ==
  NavMode : Inport
  Add : Sum  Inputs=-+
  Compare To Constant : simulink/Logic and Bit Operations/Compare To Constant  relop===  const=1  OutDataTypeStr=boolean  ZeroCross=off
  Constant : Constant
  Data Type Conversion : DataTypeConversion  OutDataTypeStr=double
  Gain : Gain  Gain=0.6
  Radar : Outport  VectorParamsAs1DForOutWhenUnconnected=off
  wires:
  NavMode/1 -> Compare To Constant/1
  Compare To Constant/1 -> Data Type Conversion/1
  Data Type Conversion/1 -> Gain/1
  Gain/1 -> Add/1
  Constant/1 -> Add/2
  Add/1 -> Radar/1

== system asbCubeSat/Visualization/Virtual Reality World/Sat Position to VRML ==
  x : Inport
  ECEF to VRML : Subsystem
  Length Conversion : aerolibconvert2/Length Conversion  IU=m  OU=km
  km to VRML units : Gain  Gain=1/1000
  xVRML : Outport  VectorParamsAs1DForOutWhenUnconnected=off
  wires:
  ECEF to VRML/1(VR) -> xVRML/1
  x/1 -> Length Conversion/1
  km to VRML units/1 -> ECEF to VRML/1(M)
  Length Conversion/1 -> km to VRML units/1

== system asbCubeSat/Visualization/Virtual Reality World/Satellite Model Scaling ==
  Constant : Constant  Value=cubesatSize
  Mux : Mux  Inputs=3
  ScaleModelToVRML : Gain  Gain=1/.3e6
  Out1 : Outport  VectorParamsAs1DForOutWhenUnconnected=off
  wires:
  ScaleModelToVRML/1 -> Mux/3, Mux/1, Mux/2
  Constant/1 -> ScaleModelToVRML/1
  Mux/1 -> Out1/1

== system asbCubeSat/Visualization/Virtual Reality World/Sun Position to VRML ==
  x : Inport
  ECEF to VRML : Subsystem
  Length Conversion : aerolibconvert2/Length Conversion  IU=m  OU=km
  km to VRML units : Gain  Gain=1/1000
  xVRML : Outport  VectorParamsAs1DForOutWhenUnconnected=off
  wires:
  ECEF to VRML/1(VR) -> xVRML/1
  x/1 -> Length Conversion/1
  km to VRML units/1 -> ECEF to VRML/1(M)
  Length Conversion/1 -> km to VRML units/1

== system asbCubeSat/Visualization/Virtual Reality World/Antenna Position to VRML/ECEF to VRML ==
  M : Inport  PortDimensions=3
  Selector : Selector  InputPortWidth=3  IndexOptions=Index vector (dialog)  Indices=[2 3 1]  OutputSizes=1
  VR : Outport  PortDimensions=3  VectorParamsAs1DForOutWhenUnconnected=off
  wires:
  M/1 -> Selector/1
  Selector/1 -> VR/1

== system asbCubeSat/Visualization/Virtual Reality World/Compute Earth Rotation Rate/Quaternion to VRML ==
  q : Inport
  Demux : Demux
  Gain : Gain  Gain=2
  Gain3 : Gain  Gain=[-1 1 1 1]
  Mux : Mux
  Selector : Selector  InputPortWidth=4  IndexOptions=Index vector (dialog)  Indices=[2 4 3 1]  OutputSizes=1
  Trigonometric Function : Trigonometry  Operator=acos
  AxisAngle : Outport  VectorParamsAs1DForOutWhenUnconnected=off
  wires:
  Demux/4 -> Mux/4
  Demux/3 -> Mux/3
  Demux/2 -> Mux/2
  Gain/1 -> Mux/1
  Selector/1 -> Gain3/1
  Gain3/1 -> AxisAngle/1
  q/1 -> Demux/1
  Mux/1 -> Selector/1
  Trigonometric Function/1 -> Gain/1
  Demux/1 -> Trigonometric Function/1

== system asbCubeSat/Visualization/Virtual Reality World/Compute Umbra Translation/unitVec ==
  I : Inport
  Divide : Product  Inputs=*/
  Dot Product : DotProduct  InputSameDT=on  OutDataTypeStr=Inherit: Inherit via internal rule
  Sqrt : Sqrt  SaturateOnIntegerOverflow=on
  O : Outport  VectorParamsAs1DForOutWhenUnconnected=off
  wires:
  Dot Product/1 -> Sqrt/1
  I/1 -> Divide/1, Dot Product/1, Dot Product/2
  Divide/1 -> O/1
  Sqrt/1 -> Divide/2

== system asbCubeSat/Visualization/Virtual Reality World/Sat Position to VRML/ECEF to VRML ==
  M : Inport  PortDimensions=3
  Selector : Selector  InputPortWidth=3  IndexOptions=Index vector (dialog)  Indices=[2 3 1]  OutputSizes=1
  VR : Outport  PortDimensions=3  VectorParamsAs1DForOutWhenUnconnected=off
  wires:
  M/1 -> Selector/1
  Selector/1 -> VR/1

== system asbCubeSat/Visualization/Virtual Reality World/Sun Position to VRML/ECEF to VRML ==
  M : Inport  PortDimensions=3
  Selector : Selector  InputPortWidth=3  IndexOptions=Index vector (dialog)  Indices=[2 3 1]  OutputSizes=1
  VR : Outport  PortDimensions=3  VectorParamsAs1DForOutWhenUnconnected=off
  wires:
  M/1 -> Selector/1
  Selector/1 -> VR/1

== matlab function asbCubeSat/Vehicle Model/Subsystem/Subsystem1/MATLAB Function ==
  data: u input; y output
function y = skew(u)

y = [0 -u(3) u(2);
    u(3) 0 -u(1);
    -u(2) u(1) 0];
